simulink model "Impedance"  (R2023b)
settings: Solver=VariableStepAuto  StartTime=0.0  StopTime=10.0  RelTol=1e-3
values from neighbouring files (symbols this model uses):
  B = 1.36e-6    (= 1.36e-06)    [Admittance_code.m]    (also in motor_model_state_space.m = [0 ; 0 ; 1/L])
  D = [0]    [motor_model_state_space.m]
  K = 1.10e-4    (= 0.00011)    [Admittance_code.m]    (also in motor_model_state_space.m = 100)
  M_inv = 1/J    (= 617283.950617)    [Admittance_code.m]    (also in motor_model_state_space.m = 1000000)
settings Model: Creator=sayeholoumi  LastModifiedBy=sayeholoumi

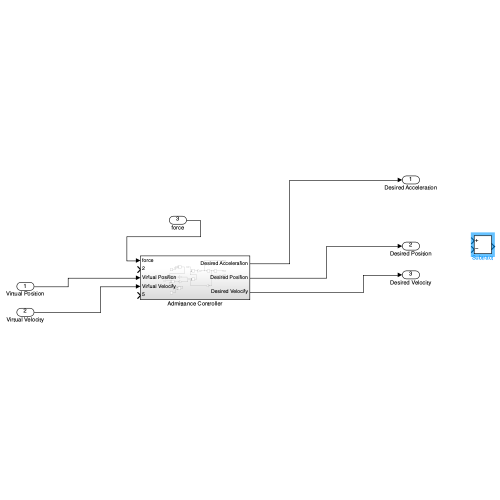
[thumbnail: Simulink's stored preview of the top-level diagram]
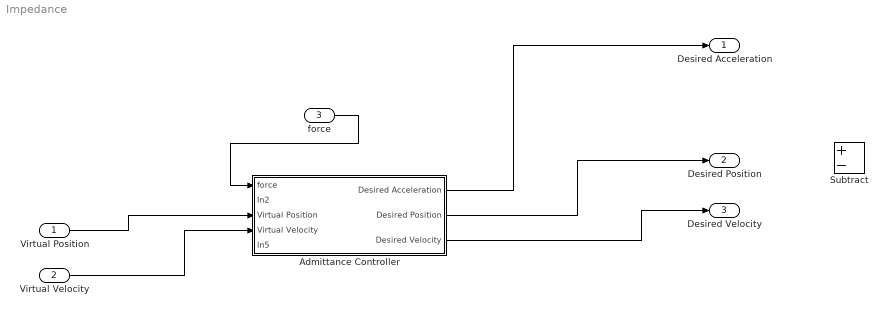
== system Impedance ==
  Virtual Position : Inport
  Virtual Velocity : Inport  Port=2
  force : Inport  Port=3
  Admittance Controller : Subsystem
  Subtract : Sum  Inputs=+-
  Desired Acceleration : Outport
  Desired Position : Outport  Port=2
  Desired Velocity : Outport  Port=3
  wires:
  force/1 -> Admittance Controller/1(force)
  Virtual Position/1 -> Admittance Controller/3(Virtual Position)
  Virtual Velocity/1 -> Admittance Controller/4(Virtual Velocity)
  Admittance Controller/1(Desired Acceleration) -> Desired Acceleration/1
  Admittance Controller/2(Desired Position) -> Desired Position/1
  Admittance Controller/3(Desired Velocity) -> Desired Velocity/1

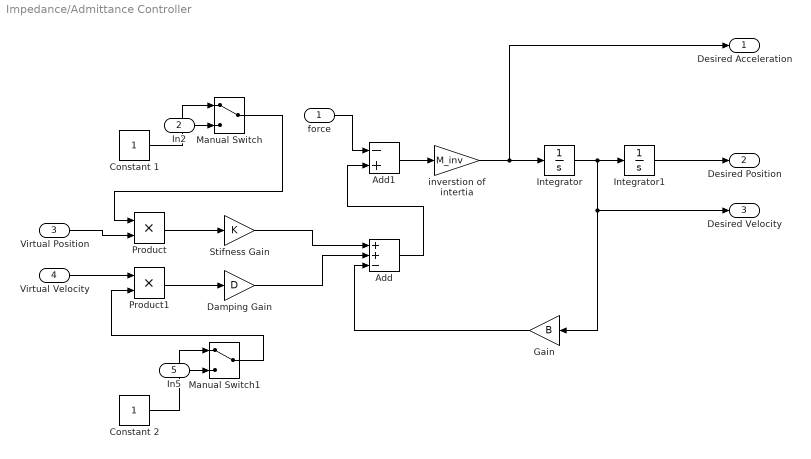
== system Impedance/Admittance Controller ==
  force : Inport
  In2 : Inport  Port=2
  Virtual Position : Inport  Port=3
  Virtual Velocity : Inport  Port=4
  In5 : Inport  Port=5
  Add : Sum  Inputs=++-
  Add1 : Sum  Inputs=-+
  Constant 1 : Constant
  Constant 2 : Constant
  Damping Gain : Gain  Gain=D
  Gain : Gain  Gain=B
  Integrator : Integrator
  Integrator1 : Integrator
  Manual Switch : ManualSwitch
  Manual Switch1 : ManualSwitch
  Product : Product
  Product1 : Product
  Stifness Gain : Gain  Gain=K
  inverstion of intertia : Gain  Gain=M_inv
  Desired Acceleration : Outport
  Desired Position : Outport  Port=2
  Desired Velocity : Outport  Port=3
  wires:
  In5/1 -> Manual Switch1/2
  In2/1 -> Manual Switch/2
  Manual Switch1/1 -> Product1/2
  Constant 2/1 -> Manual Switch1/1
  Add1/1 -> inverstion of intertia/1
  Integrator/1 -> Desired Velocity/1, Gain/1, Integrator1/1
  Constant 1/1 -> Manual Switch/1
  Product/1 -> Stifness Gain/1
  Gain/1 -> Add/3
  Stifness Gain/1 -> Add/1
  Integrator1/1 -> Desired Position/1
  Virtual Position/1 -> Product/2
  Damping Gain/1 -> Add/2
  force/1 -> Add1/1
  Add/1 -> Add1/2
  inverstion of intertia/1 -> Desired Acceleration/1, Integrator/1
  Manual Switch/1 -> Product/1
  Product1/1 -> Damping Gain/1
  Virtual Velocity/1 -> Product1/1
